simulink model "g03_CommTx"  (R2024a)
settings: Solver=FixedStepDiscrete  StartTime=0.0  StopTime=1  FixedStep=mSim.dTime  MaxStep=Define.sModelSampleTime  RelTol=7.1420e-05
undefined symbols (not defined in the file): CTX3
libraries: simulink x5, hdlsllib x3
settings Model: Creator=user  LastModifiedBy=admin
settings SolverCC: MaxConsecutiveZCs=10000  ZeroCrossAlgorithm=Adaptive  AlgebraicLoopSolver=TrustRegion
settings DataIOCC: SaveOutput=off  DSMLogging=off  InspectSignalLogs=on  SaveTime=off  SignalLoggingName=logsout_Validator
settings OptimizationCC: BlockReduction=off  DefaultParameterBehavior=Inlined  UseDivisionForNetSlopeComputation=UseDivisionForReciprocalsOfIntegersOnly  GainParamInheritBuiltInType=on  UseFloatMulNetSlope=on  DefaultUnderspecifiedDataType=single  InlineInvariantSignals=on  BitwiseOrLogicalOp=Logical operator  PassReuseOutputArgsAs=Individual arguments  EfficientFloat2IntCast=on  LifeSpan=Inf  OptimizeBlockOrder=speed  DifferentSizesBufferReuse=on  EfficientTunableParamExpr=on
settings DebuggingCC: SignalInfNanChecking=error  SignalRangeChecking=error  ReadBeforeWriteMsg=EnableAllAsError  WriteAfterWriteMsg=EnableAllAsError  WriteAfterReadMsg=EnableAllAsError  AlgebraicLoopMsg=error  ArtificialAlgebraicLoopMsg=error  SaveWithDisabledLinksMsg=error  SaveWithParameterizedLinksMsg=error  BlockPriorityViolationMsg=error  SolverPrmCheckMsg=error  InheritedTsInSrcMsg=error  SingleTaskRateTransMsg=error  TasksWithSamePriorityMsg=error  SigSpecEnsureSampleTimeMsg=error  CheckMatrixSingularityMsg=error  IntegerOverflowMsg=error  ParameterUnderflowMsg=error  ParameterPrecisionLossMsg=error  ParameterTunabilityLossMsg=error  UnderSpecifiedDataTypeMsg=error  UnnecessaryDatatypeConvMsg=warning  VectorMatrixConversionMsg=error  SignalLabelMismatchMsg=error  UnconnectedInputMsg=error  UnconnectedOutputMsg=error  UnconnectedLineMsg=error  SFcnCompatibilityMsg=error  UniqueDataStoreMsg=error  BusObjectLabelMismatch=error  RootOutportRequireBusObject=error  AssertControl=DisableAll  ModelReferenceIOMismatchMessage=error  UnknownTsInhSupMsg=error  ModelReferenceDataLoggingMessage=error  ModelReferenceSymbolNameMessage=none  StateNameClashWarn=warning  StrictBusMsg=ErrorOnBusTreatedAsVector  NonBusSignalsTreatedAsBus=error  SFInvalidInputDataAccessInChartInitDiag=error  SFTransitionOutsideNaturalParentDiag=error  SFUnreachableExecutionPathDiag=error  SFUndirectedBroadcastEventsDiag=error  SFTransitionActionBeforeConditionDiag=error  SFTemporalDelaySmallerThanSampleTimeDiag=error  SFSelfTransitionDiag=error  SFExecutionAtInitializationDiag=error  IntegerSaturationMsg=error  UnitsInconsistencyMsg=none  VariantConditionMismatch=error
settings HardwareCC: ProdBitPerChar=16  ProdBitPerInt=16  ProdBitPerPointer=32  ProdBitPerSizeT=32  ProdBitPerPtrDiffT=32  ProdLargestAtomicInteger=Integer  ProdLargestAtomicFloat=None  ProdWordSize=16  ProdLongLongMode=on  ProdHWDeviceType=Texas Instruments->C2000
settings ModelReferenceCC: EnableRefExpFcnMdlSchedulingChecks=on  ModelReferenceNumInstancesAllowed=Single
settings SFSimCC: SimUseLocalCustomCode=off  CompileTimeRecursionLimit=0  EnableRuntimeRecursion=off  MATLABDynamicMemAlloc=off  CustomCodeUndefinedFunction=UseInterfaceOnly
settings RTWCC: Description=Embedded Coder  SystemTargetFile=ert.tlc  GenCodeOnly=on  TemplateMakefile=ert_default_tmf  GenerateReport=on  RTWUseLocalCustomCode=off  CustomInitializer=mM2Int_SwRev = CTX3.uSW_REV;  BuildConfiguration=Faster Runs  IncludeHyperlinkInReport=on  LaunchReport=on  GenerateTraceInfo=on  GenerateTraceReport=on  GenerateTraceReportSl=on  GenerateTraceReportSf=on  GenerateWebview=on  GenerateCodeMetricsReport=on  GenerateCodeReplacementReport=on  GPUComputeCapability=3.5  DLArmComputeVersion=19.05
settings CodeAppCC: ForceParamTrailComments=on  IgnoreCustomStorageClasses=off  MATLABFcnDesc=on  MangleLength=4  CustomSymbolStrGlobalVar=GvG03$N$M  CustomSymbolStrType=StrG03$N$M  CustomSymbolStrFcn=$N$M$F  CustomSymbolStrMacro=$N$M  DefineNamingRule=UpperCase  ParamNamingRule=UpperCase  SimulinkBlockComments=off  MATLABSourceComments=on  EnableCustomComments=on  ReqsInCode=on
settings ERTTargetCC: TargetLangStandard=C99 (ISO)  UtilityFuncGeneration=Shared location  MultiwordLength=2048  IncludeMdlTerminateFcn=off  CombineSignalStateStructs=on  SuppressErrorStatus=on  SupportAbsoluteTime=off  SupportNonFinite=off  ParenthesesLevel=Maximum  CastingMode=Standards  GenerateSharedConstants=off  InlinedParameterPlacement=NonHierarchical  ERTSrcFileBannerTemplate=t_code_template.cgt  ERTHdrFileBannerTemplate=t_code_template.cgt  ERTDataSrcFileTemplate=t_code_template.cgt  ERTDataHdrFileTemplate=t_code_template.cgt  ERTCustomFileTemplate=example_file_process.tlc  ERTFilePackagingFormat=CompactWithDataFile  PreserveExpressionOrder=on  SuppressUnreachableDefaultCases=off  EnableSignedLeftShifts=off  EnableSignedRightShifts=off  IndentStyle=Allman  IndentSize=4
settings ConfigComp: CovSaveName=coveragedata  CovMetricSettings=we  CovEnableCumulative=off  CovSaveCumulativeToWorkspaceVar=on  CovSaveSingleToWorkspaceVar=on  CovOutputDir=sldv_output/$ModelName$\sldv_covoutput  PSVerificationMode=BugFinder  PSModelRefIgnoreList=[]  PSEnableModelRefIgnoreList=off  PSModelRefMinMaxVerif=CheckAndConstrain  PSAutoStubLUT=on  DVModelCoverageObjectives=MCDC  DVTestSuiteOptimization=CombinedObjectives (Nonlinear Extended)  DVRebuildModelRepresentation=Always
settings SimscapeCC: SimscapeNormalizeSystem=off

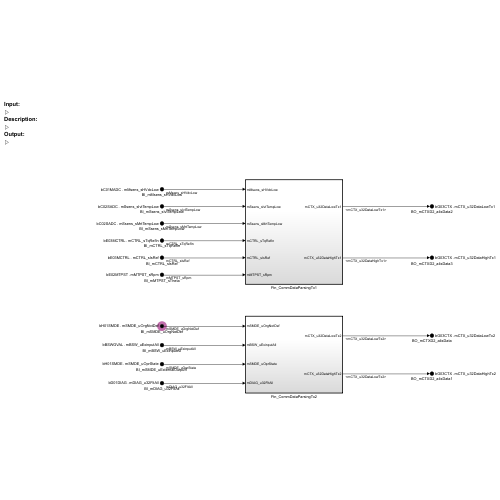
[thumbnail: Simulink's stored preview of the top-level diagram]
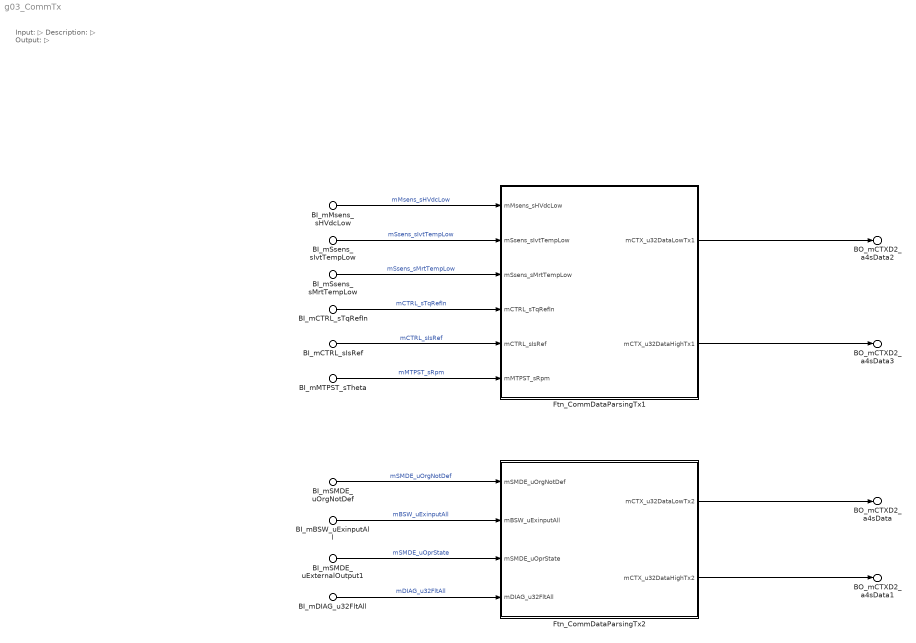
== system g03_CommTx ==
  note: Input:
      | ▷
      | Description:
      | ▷
      | Output:
      | ▷
  BI_mSMDE_uExternalOutput1 : Inport  Description=■ 설명: 운영 모드 (1H : Standby / 2H : JOG / 4H : MPG_JOG / 8H: Operating / 16H : Wait / 32H: Origin)  PortName=bH01SMDE  Element=mSMDE_uOprState
  BI_mSMDE_uOrgNotDef : Inport  Description=■ 설명: 원점 설정 유무를 나타내는 출력입니다. (ON: 원점 설정 없음, OFF: 원점 설정), 통신용  PortName=bH01SMDE  Element=mSMDE_uOrgNotDef
  BI_mDIAG_u32FltAll : Inport  Description=■ 설명: 고장 신호 전체값  Port=2  PortName=bD01DIAG  Element=mDIAG_u32FltAll
  BI_mMsens_sHVdcLow : Inport  Description=■ 설명: DC Link 전압  Port=3  PortName=bC01MADC  Element=mMsens_sHVdcLow
  BI_mSsens_sIvtTempLow : Inport  Description=■ 설명: IGBT 온도  Port=4  PortName=bC02SADC  Element=mSsens_sIvtTempLow
  BI_mSsens_sMrtTempLow : Inport  Description=■ 설명: 모터 온도  Port=4  PortName=bC02SADC  Element=mSsens_sMrtTempLow
  BI_mCTRL_sIsRef : Inport  Description=■ 설명: Is 전류 지령  Port=5  PortName=bE03MCTRL  Element=mCTRL_sIsRef
  BI_mCTRL_sTqRefIn : Inport  Description=■ 설명: 토크 지령  Port=5  PortName=bE03MCTRL  Element=mCTRL_sTqRefIn
  BI_mMTPST_sTheta : Inport  Description=■ 설명: Motor Speed  Port=6  PortName=bE02MTPST  Element=mMTPST_sRpm
  BI_mBSW_uExinputAll : Inport  Description=■ 설명: Digital Input Signal  Port=7  PortName=bBSWGVAL  Element=mBSW_uExinputAll
  Ftn_CommDataParsingTx1 : Subsystem  TreatAsAtomicUnit=on
      settings: RTWSystemCode=Nonreusable function  RTWFcnNameOpts=Use subsystem name
  Ftn_CommDataParsingTx2 : Subsystem  TreatAsAtomicUnit=on
      settings: RTWSystemCode=Nonreusable function  RTWFcnNameOpts=Use subsystem name
  BO_mCTXD2_a4sData2 : Outport  Description=■ 설명: 통신 TX1 Low 32Bit  PortName=bG03CTX  Element=mCTX_u32DataLowTx1
  BO_mCTXD2_a4sData3 : Outport  Description=■ 설명: 통신 TX1 Higt 32Bit  PortName=bG03CTX  Element=mCTX_u32DataHighTx1
  BO_mCTXD2_a4sData : Outport  Description=■ 설명: 통신 TX2 Low 32Bit  PortName=bG03CTX  Element=mCTX_u32DataLowTx2
  BO_mCTXD2_a4sData1 : Outport  Description=■ 설명: 통신 TX2 Higt 32Bit  PortName=bG03CTX  Element=mCTX_u32DataHighTx2
  wires:
  BI_mSMDE_uOrgNotDef/1 -> Ftn_CommDataParsingTx2/1(mSMDE_uOrgNotDef)  "mSMDE_uOrgNotDef"
  BI_mDIAG_u32FltAll/1 -> Ftn_CommDataParsingTx2/4(mDIAG_u32FltAll)  "mDIAG_u32FltAll"
  Ftn_CommDataParsingTx2/1(mCTX_u32DataLowTx2) -> BO_mCTXD2_a4sData/1
  Ftn_CommDataParsingTx2/2(mCTX_u32DataHighTx2) -> BO_mCTXD2_a4sData1/1
  BI_mMsens_sHVdcLow/1 -> Ftn_CommDataParsingTx1/1(mMsens_sHVdcLow)  "mMsens_sHVdcLow"
  BI_mSsens_sIvtTempLow/1 -> Ftn_CommDataParsingTx1/2(mSsens_sIvtTempLow)  "mSsens_sIvtTempLow"
  BI_mSsens_sMrtTempLow/1 -> Ftn_CommDataParsingTx1/3(mSsens_sMrtTempLow)  "mSsens_sMrtTempLow"
  BI_mCTRL_sTqRefIn/1 -> Ftn_CommDataParsingTx1/4(mCTRL_sTqRefIn)  "mCTRL_sTqRefIn"
  BI_mCTRL_sIsRef/1 -> Ftn_CommDataParsingTx1/5(mCTRL_sIsRef)  "mCTRL_sIsRef"
  BI_mMTPST_sTheta/1 -> Ftn_CommDataParsingTx1/6(mMTPST_sRpm)  "mMTPST_sRpm"
  Ftn_CommDataParsingTx1/1(mCTX_u32DataLowTx1) -> BO_mCTXD2_a4sData2/1
  Ftn_CommDataParsingTx1/2(mCTX_u32DataHighTx1) -> BO_mCTXD2_a4sData3/1
  BI_mSMDE_uExternalOutput1/1 -> Ftn_CommDataParsingTx2/3(mSMDE_uOprState)  "mSMDE_uOprState"
  BI_mBSW_uExinputAll/1 -> Ftn_CommDataParsingTx2/2(mBSW_uExinputAll)  "mBSW_uExinputAll"

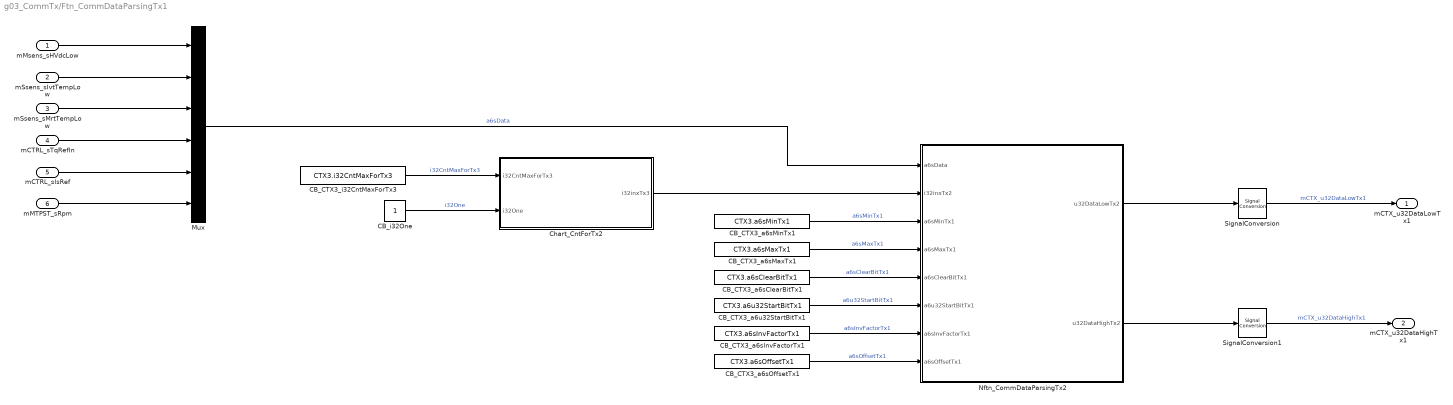
== system g03_CommTx/Ftn_CommDataParsingTx1 ==
  mMsens_sHVdcLow : Inport
  mSsens_sIvtTempLow : Inport  Port=2
  mSsens_sMrtTempLow : Inport  Port=3
  mCTRL_sTqRefIn : Inport  Port=4
  mCTRL_sIsRef : Inport  Port=5
  mMTPST_sRpm : Inport  Port=6
  CB_CTX3_a6sClearBitTx1 : Constant  Value=CTX3.a6sClearBitTx1
  CB_CTX3_a6sInvFactorTx1 : Constant  Value=CTX3.a6sInvFactorTx1
  CB_CTX3_a6sMaxTx1 : Constant  Value=CTX3.a6sMaxTx1
  CB_CTX3_a6sMinTx1 : Constant  Value=CTX3.a6sMinTx1
  CB_CTX3_a6sOffsetTx1 : Constant  Value=CTX3.a6sOffsetTx1
  CB_CTX3_a6u32StartBitTx1 : Constant  Value=CTX3.a6u32StartBitTx1
  CB_CTX3_i32CntMaxForTx3 : Constant  Value=CTX3.i32CntMaxForTx3  OutDataTypeStr=int32
  CB_i32One : Constant  OutDataTypeStr=int32
  Chart_CntForTx2 : Stateflow chart  TreatAsAtomicUnit=on
  Mux : Mux  Inputs=6
  Nftn_CommDataParsingTx2 : Stateflow chart  RTWFcnName=ftn_CommChartDataParsing
      settings: RTWSystemCode=Nonreusable function  RTWFcnNameOpts=Use subsystem name
  SignalConversion : SignalConversion  OverrideOpt=off
  SignalConversion1 : SignalConversion  OverrideOpt=off
  mCTX_u32DataLowTx1 : Outport
  mCTX_u32DataHighTx1 : Outport  Port=2
  wires:
  mCTRL_sIsRef/1 -> Mux/5
  Mux/1 -> Nftn_CommDataParsingTx2/1(a6sData)  "a6sData"
  mSsens_sMrtTempLow/1 -> Mux/3
  mCTRL_sTqRefIn/1 -> Mux/4
  mMTPST_sRpm/1 -> Mux/6
  mMsens_sHVdcLow/1 -> Mux/1
  mSsens_sIvtTempLow/1 -> Mux/2
  CB_CTX3_a6sInvFactorTx1/1 -> Nftn_CommDataParsingTx2/7(a6sInvFactorTx1)  "a6sInvFactorTx1"
  CB_CTX3_i32CntMaxForTx3/1 -> Chart_CntForTx2/1(i32CntMaxForTx3)  "i32CntMaxForTx3"
  CB_i32One/1 -> Chart_CntForTx2/2(i32One)  "i32One"
  CB_CTX3_a6sClearBitTx1/1 -> Nftn_CommDataParsingTx2/5(a6sClearBitTx1)  "a6sClearBitTx1"
  Nftn_CommDataParsingTx2/1(u32DataLowTx2) -> SignalConversion/1
  CB_CTX3_a6sMaxTx1/1 -> Nftn_CommDataParsingTx2/4(a6sMaxTx1)  "a6sMaxTx1"
  CB_CTX3_a6sOffsetTx1/1 -> Nftn_CommDataParsingTx2/8(a6sOffsetTx1)  "a6sOffsetTx1"
  CB_CTX3_a6u32StartBitTx1/1 -> Nftn_CommDataParsingTx2/6(a6u32StartBitTx1)  "a6u32StartBitTx1"
  CB_CTX3_a6sMinTx1/1 -> Nftn_CommDataParsingTx2/3(a6sMinTx1)  "a6sMinTx1"
  Chart_CntForTx2/1(i32inxTx3) -> Nftn_CommDataParsingTx2/2(i32inxTx2)
  Nftn_CommDataParsingTx2/2(u32DataHighTx2) -> SignalConversion1/1
  SignalConversion1/1 -> mCTX_u32DataHighTx1/1  "mCTX_u32DataHighTx1"
  SignalConversion/1 -> mCTX_u32DataLowTx1/1  "mCTX_u32DataLowTx1"

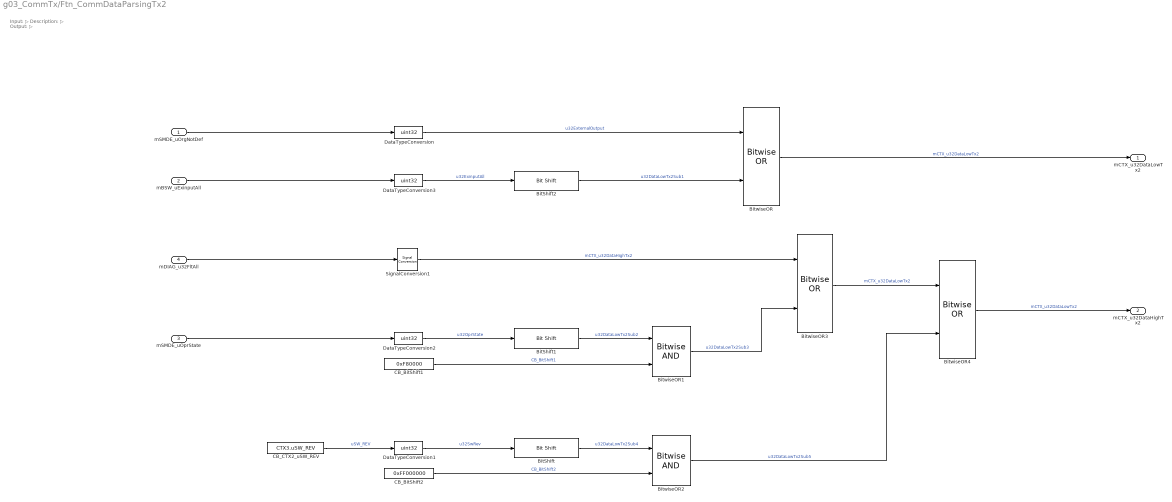
== system g03_CommTx/Ftn_CommDataParsingTx2 ==
  note: Input:
      | ▷
      | Description:
      | ▷
      | Output:
      | ▷
  mSMDE_uOrgNotDef : Inport
      settings: AttributesFormatString=|
      | ■ SWC Name: %<Parent>
      | ■ DataType: uint32
      | ■ Max: %<OutMax>
      | ■ Min: %<OutMin>
      | %<Description>
  mBSW_uExinputAll : Inport  Port=2
      settings: AttributesFormatString=|
      | ■ SWC Name: %<Parent>
      | ■ DataType: uint32
      | ■ Max: %<OutMax>
      | ■ Min: %<OutMin>
      | %<Description>
  mSMDE_uOprState : Inport  Port=3
      settings: AttributesFormatString=|
      | ■ SWC Name: %<Parent>
      | ■ DataType: uint32
      | ■ Max: %<OutMax>
      | ■ Min: %<OutMin>
      | %<Description>
  mDIAG_u32FltAll : Inport  Port=4
      settings: AttributesFormatString=|
      | ■ SWC Name: %<Parent>
      | ■ DataType: uint32
      | ■ Max: %<OutMax>
      | ■ Min: %<OutMin>
      | %<Description>
  BitShift : hdlsllib/Logic and Bit Operations/Bit Shift  mode=Shift Left Logical  N=24
  BitShift1 : hdlsllib/Logic and Bit Operations/Bit Shift  mode=Shift Left Logical  N=19
  BitShift2 : hdlsllib/Logic and Bit Operations/Bit Shift  mode=Shift Left Logical  N=16
  BitwiseOR : simulink/Logic and Bit Operations/Bitwise Operator  logicop=OR  UseBitMask=off  NumInputPorts=2  BitMask=bin2dec('11011001')  BitMaskRealWorld=Stored Integer
      settings: LibrarySourceBlock=|
      | simulink/Quick Insert/Logic and Bit
      | Operations/Bitwise OR
  BitwiseOR1 : simulink/Logic and Bit Operations/Bitwise Operator  logicop=AND  UseBitMask=off  NumInputPorts=2  BitMask=bin2dec('11011001')  BitMaskRealWorld=Stored Integer
      settings: LibrarySourceBlock=|
      | simulink/Quick Insert/Logic and Bit
      | Operations/Bitwise OR
  BitwiseOR2 : simulink/Logic and Bit Operations/Bitwise Operator  logicop=AND  UseBitMask=off  NumInputPorts=2  BitMask=bin2dec('11011001')  BitMaskRealWorld=Stored Integer
      settings: LibrarySourceBlock=|
      | simulink/Quick Insert/Logic and Bit
      | Operations/Bitwise OR
  BitwiseOR3 : simulink/Logic and Bit Operations/Bitwise Operator  logicop=OR  UseBitMask=off  NumInputPorts=2  BitMask=bin2dec('11011001')  BitMaskRealWorld=Stored Integer
      settings: LibrarySourceBlock=|
      | simulink/Quick Insert/Logic and Bit
      | Operations/Bitwise OR
  BitwiseOR4 : simulink/Logic and Bit Operations/Bitwise Operator  logicop=OR  UseBitMask=off  NumInputPorts=2  BitMask=bin2dec('11011001')  BitMaskRealWorld=Stored Integer
      settings: LibrarySourceBlock=|
      | simulink/Quick Insert/Logic and Bit
      | Operations/Bitwise OR
  CB_BitShift1 : Constant  Value=0xF80000  OutDataTypeStr=uint32
  CB_BitShift2 : Constant  Value=0xFF000000  OutDataTypeStr=uint32
  CB_CTX2_uSW_REV : Constant  Value=CTX3.uSW_REV
  DataTypeConversion{,1..3} (4 alike) : DataTypeConversion  OutDataTypeStr=uint32  SaturateOnIntegerOverflow=off  RndMeth=Floor
  SignalConversion1 : SignalConversion  OverrideOpt=off
  mCTX_u32DataLowTx2 : Outport
      settings: AttributesFormatString=|
      | ■ SWC Name: %<Parent>
      | ■ DataType: uint32
      | ■ Max: %<OutMax>
      | ■ Min: %<OutMin>
      | %<Description>
  mCTX_u32DataHighTx2 : Outport  Description=■ 설명: mCTX1_u32TxHigh  Port=2  OutMin=0  OutMax=4294967295
      settings: AttributesFormatString=|
      | ■ SWC Name: %<Parent>
      | ■ DataType: uint32
      | ■ Max: %<OutMax>
      | ■ Min: %<OutMin>
      | %<Description>
  wires:
  BitShift/1 -> BitwiseOR2/1  "u32DataLowTx2Sub4"
  CB_CTX2_uSW_REV/1 -> DataTypeConversion1/1  "uSW_REV"
  SignalConversion1/1 -> BitwiseOR3/1  "mCTX_u32DataHighTx2"
  mDIAG_u32FltAll/1 -> SignalConversion1/1
  mSMDE_uOrgNotDef/1 -> DataTypeConversion/1
  BitwiseOR/1 -> mCTX_u32DataLowTx2/1  "mCTX_u32DataLowTx2"
  DataTypeConversion/1 -> BitwiseOR/1  "u32ExternalOutput"
  DataTypeConversion1/1 -> BitShift/1  "u32SwRev"
  mSMDE_uOprState/1 -> DataTypeConversion2/1
  DataTypeConversion2/1 -> BitShift1/1  "u32OprState"
  BitShift1/1 -> BitwiseOR1/1  "u32DataLowTx2Sub2"
  CB_BitShift1/1 -> BitwiseOR1/2  "CB_BitShift1"
  BitwiseOR1/1 -> BitwiseOR3/2  "u32DataLowTx2Sub3"
  CB_BitShift2/1 -> BitwiseOR2/2  "CB_BitShift2"
  BitwiseOR2/1 -> BitwiseOR4/2  "u32DataLowTx2Sub5"
  mBSW_uExinputAll/1 -> DataTypeConversion3/1
  DataTypeConversion3/1 -> BitShift2/1  "u32ExinputAll"
  BitShift2/1 -> BitwiseOR/2  "u32DataLowTx2Sub1"
  BitwiseOR3/1 -> BitwiseOR4/1  "mCTX_u32DataLowTx2"
  BitwiseOR4/1 -> mCTX_u32DataHighTx2/1  "mCTX_u32DataLowTx2"

== stateflow chart g03_CommTx/Ftn_CommDataParsingTx1/Nftn_CommDataParsingTx2 ==
  (default) -> (junction 509)
  (junction 509) -> (junction 510) [order 1] : [a6sData[i32inxTx2] >= a6sMaxTx1[i32inxTx2]]
  (junction 509) -> (junction 553) [order 2]
  (junction 510) -> (junction 512) : {
      | sTxData = a6sMaxTx1[i32inxTx2];
      | }
  (junction 553) -> (junction 552) [order 1] : [a6sData[i32inxTx2] <= a6sMinTx1[i32inxTx2]]
  (junction 553) -> (junction 550) [order 2] : {
      | sTxData = a6sData[i32inxTx2];
      | }
  (junction 552) -> (junction 554) : {
      | sTxData = a6sMinTx1[i32inxTx2];
      | }
  (junction 554) -> (junction 550)
  (junction 512) -> (junction 554)
  (junction 550) -> (junction 358) : {
      | a32u32TxData = uint32(((sTxData - a6sOffsetTx1[i32inxTx2]) * a6sInvFactorTx1[i32inxTx2]));
      | }
  (junction 358) -> (junction 359) [order 1] : [a6u32StartBitTx1[i32inxTx2] >= Cnst_u32_32]
  (junction 358) -> (junction 534) [order 2]
  (junction 359) -> (junction 543)
  (junction 534) -> (junction 529) [order 1] : [a6u32StartBitTx1[i32inxTx2] == Cnst_u32_0]
  (junction 543) -> (junction 541) [order 1] : [a6u32StartBitTx1[i32inxTx2] == Cnst_u32_32]
  (junction 534) -> (junction 528) [order 2] : {
      | Local_u32LowOut = a32u32TxData<<a6u32StartBitTx1[i32inxTx2];
      | }
  (junction 529) -> (junction 530) : {
      | Local_u32LowOut = a32u32TxData;
      | }
  (junction 543) -> (junction 542) [order 2] : {
      | Local_u32HighOut = a32u32TxData << (a6u32StartBitTx1[i32inxTx2] - Cnst_u32_32);
      | }
  (junction 541) -> (junction 537) : {
      | Local_u32HighOut = a32u32TxData;
      | }
  (junction 530) -> (junction 528)
  (junction 537) -> (junction 542)
  (junction 528) -> (junction 401) : {
      | u32DataLowTx2 &= a6sClearBitTx1[i32inxTx2];
      | u32DataLowTx2 |= Local_u32LowOut;
      | }
  (junction 542) -> (junction 364) : /* Spare bit is always set to 1. (The initial value of u32DataHighTx2 is set to 0x80000000.)*/
      | {
      | u32DataHighTx2 &= a6sClearBitTx1[i32inxTx2];
      | u32DataHighTx2 |= Local_u32HighOut;
      | }
  (junction 364) -> (junction 401)
  (junction 401) -> (junction 484)
  data: a6sData input; i32inxTx2 input; a6sMinTx1 input; a6sMaxTx1 input; a6sClearBitTx1 input; a6u32StartBitTx1 input; a6sInvFactorTx1 input; a6sOffsetTx1 input; a32u32TxData local uint32; u32DataLowTx2 output uint32; u32DataHighTx2 output uint32; sTxData local single; Local_u32LowOut local uint32; Local_u32HighOut local uint32; Cnst_u32_32 constant uint32 =32; Cnst_u32_0 constant uint32 =0

== stateflow chart g03_CommTx/Ftn_CommDataParsingTx1/Chart_CntForTx2 ==
  (default) -> (junction 2)
  (junction 2) -> (junction 3) [order 1] : [i32inxTx3 >= i32CntMaxForTx3]
  (junction 2) -> (junction 13) [order 2] : {
      | i32inxTx3 = i32inxTx3 + i32One;
      | }
  (junction 3) -> (junction 4) : {
      | i32inxTx3 = ConstG01_i32InitCntForTx2;
      | }
  (junction 4) -> (junction 13)
  (junction 13) -> (junction 34)
  data: i32inxTx3 output int32; ConstG01_i32InitCntForTx2 constant int32 =0; i32CntMaxForTx3 input int32; i32One input
